simulink model "Copy_of_smlnk"  (R2024b)
settings: Solver=ode4  StartTime=0.0  StopTime=100  FixedStep=0.0001  RelTol=1e-3
model workspace (MAT data in the model file):
  Sample_Time = 0.0001
  Sig = Simulink.Signal
  Sig.Dimensions = -1
  Sig.DimensionsMode = 'auto'
  Sig.Complexity = 'auto'
  Sig.SampleTime = -1
  Sig.SamplingMode = 'auto'
  Sig.DataType = 'auto'
  Sig1 = Simulink.Signal
  Sig1.Dimensions = -1
  Sig1.DimensionsMode = 'auto'
  Sig1.Complexity = 'auto'
  Sig1.SampleTime = -1
  Sig1.SamplingMode = 'auto'
  Sig1.DataType = 'auto'
settings Model: Creator=loren  LastModifiedBy=loren
settings RTWCC: GPUComputeCapability=3.5
settings GRTTargetCC: RTWCAPISignals=on  RTWCAPIParams=on

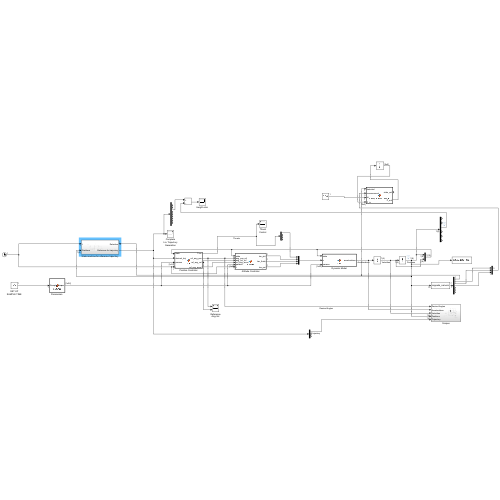
[thumbnail: Simulink's stored preview of the top-level diagram]
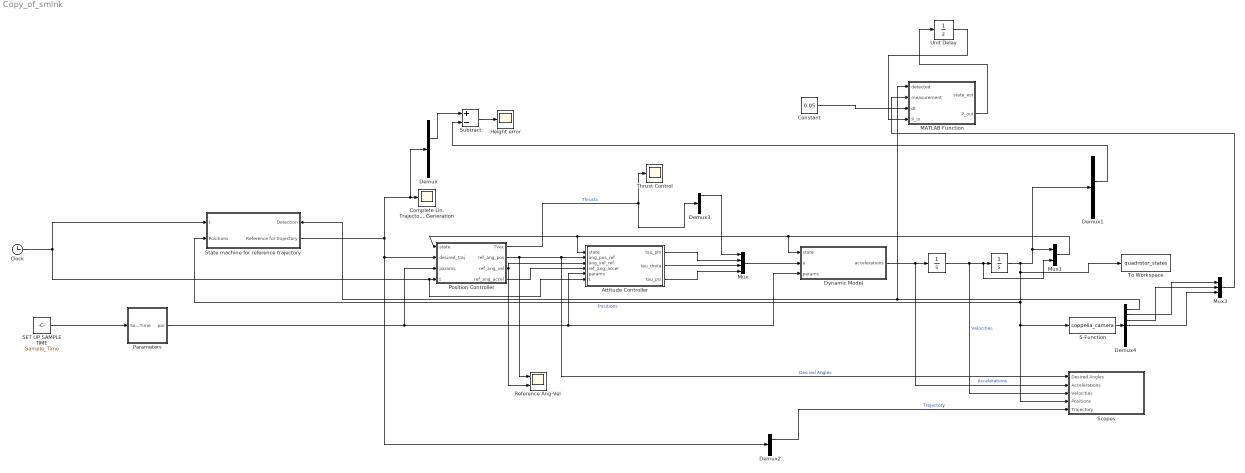
== system Copy_of_smlnk ==
  " " : Integrator  InitialCondition=[0 0 0 0 0 0]
  "  " : Integrator  InitialCondition=[0 0 0 0 0 0]
  Attitude Controller : MATLAB Function  TreatAsAtomicUnit=on  SystemSampleTime=Sample_Time
  Clock : Clock
  Complete Lin. Trajectory Generation : Scope
  Constant : Constant  Value=0.05
  Demux : Demux  Outputs=9
  Demux1 : Demux  Outputs=6
  Demux2 : Demux  Outputs=3
  Demux3 : Demux
  Demux4 : Demux  Outputs=7
  Dynamic Model : MATLAB Function  TreatAsAtomicUnit=on
  Height error : Scope
  MATLAB Function : MATLAB Function  TreatAsAtomicUnit=on
  Mux : Mux
  Mux1 : Mux  Inputs=2
  Mux3 : Mux  Inputs=3
  "Parameters " : MATLAB Function  TreatAsAtomicUnit=on  SystemSampleTime=Sample_Time
  Position Controller : MATLAB Function  TreatAsAtomicUnit=on  SystemSampleTime=Sample_Time
  Reference Ang-Vel : Scope  NumInputPorts=2
  S-Function : S-Function  FunctionName=coppelia_camera  Parameters=[Sample_Time, 1, 1]  SFunctionDeploymentMode=off  EnableBusSupport=off
  SET UP SAMPLE TIME : Constant  Value=Sample_Time
  Scopes : Subsystem
  State machine for reference trajectory : Subsystem
      settings: PortSchema="{\"entries\":[{\"content\":{\"sides\":[{\"content\":{\"connectorIds\":[\"In1\",\"In2\"]},\"type\":\"ConnectorPlacement.EquallySpacedRectSide\",\"uuid\":\"507c7cd5-8cc5-4e23-900b-3d7f1b18adf8\"},{\"content\":{\"connectorIds\":[\"In3\",\"Out1\"],\"side\":\"RIGHT\"},\"type\":\"ConnectorPlacement.EquallySpacedRectSide\",\"uuid\":\"450f9651-8ffa-4a7c-835b-1cc66628d75d\"},{\"content\":{\"side\":\"TOP\"},\"type\":\"ConnectorPlacement.EquallySpacedRectSide\",\"uuid\":\"2e914235-4cad-40eb-804a-8ecad3aa82e7\"}]},\"type\":\"ConnectorPlacement.EquallySpacedConnector\",\"uuid\":\"783284ba-16e5-4ade-a3ef-caf26ef0d258\"}],\"packageUris\":[\"http://schema.mathworks.com/mf0/Connector/R2020b\"],\"version\":\"1.0\"}"
  Subtract : Sum  Inputs=+-
  Thrust Control : Scope
  To Workspace : ToWorkspace  VariableName=quadrotor_states  SaveFormat=Structure With Time  SampleTime=-1
  Unit Delay : UnitDelay  InitialCondition=eye(5)  SampleTime=0.05  HasFrameUpgradeWarning=on
  wires:
  "Parameters "/1(par) -> Dynamic Model/3(params), Attitude Controller/5(params), Position Controller/3(params)
  Position Controller/2(ref_ang_pos) -> Reference Ang-Vel/1, Scopes/1(Desired Angles), Attitude Controller/2(ang_pos_ref)  "Desired Angles"
  Position Controller/3(ref_ang_vel) -> Reference Ang-Vel/2, Attitude Controller/3(ang_vel_ref)
  Attitude Controller/1(tau_phi) -> Mux/2
  Attitude Controller/2(tau_theta) -> Mux/3
  Attitude Controller/3(tau_psi) -> Mux/4
  Mux/1 -> Dynamic Model/2(u)
  Dynamic Model/1(accelerations) -> Scopes/2(Accelerations), " "/1  "Accelerations"
  " "/1 -> Scopes/3(Velocities), "  "/1, Mux1/2  "Velocities"
  Mux1/1 -> Dynamic Model/1(state), Position Controller/1(state), Attitude Controller/1(state)
  Demux/3 -> Subtract/1
  Demux1/3 -> Subtract/2
  Subtract/1 -> Height error/1
  Clock/1 -> Attitude Controller/6(t), Position Controller/4(t), State machine for reference trajectory/1(t)
  "  "/1 -> S-Function/1, Scopes/4(Positions), State machine for reference trajectory/2(Positions), To Workspace/1, Demux1/1, Mux1/1  "Positions"
  SET UP SAMPLE TIME/1 -> "Parameters "/1(Sample_Time)
  Position Controller/1(Tvec) -> Thrust Control/1, Demux3/1  "Thrusts"
  Demux3/1 -> Mux/1
  Demux2/1 -> Scopes/5(Trajectory)  "Trajectory"
  State machine for reference trajectory/1(Reference for trajectory) -> Demux/1, Complete Lin. Trajectory Generation/1, Position Controller/2(desired_traj), Demux2/1
  Position Controller/4(ref_ang_accel) -> Attitude Controller/4(ref_ang_accel)
  S-Function/1 -> Demux4/1
  Demux4/1 -> MATLAB Function/1(detected), State machine for reference trajectory/3(Detection)
  Demux4/2 -> Mux3/1
  Demux4/3 -> Mux3/2
  Demux4/4 -> Mux3/3
  Mux3/1 -> MATLAB Function/2(measurement)
  Constant/1 -> MATLAB Function/3(dt)
  MATLAB Function/2(P_out) -> Unit Delay/1
  Unit Delay/1 -> MATLAB Function/4(P_in)

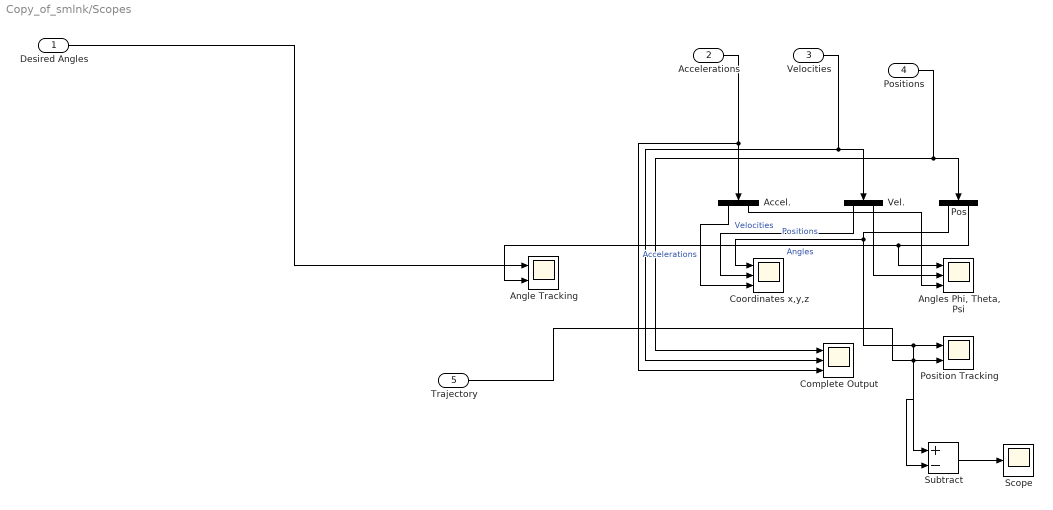
== system Copy_of_smlnk/Scopes ==
  Desired Angles : Inport
  Accelerations : Inport  Port=2
  Velocities : Inport  Port=3
  Positions : Inport  Port=4
  Trajectory : Inport  Port=5
  Accel. : Demux  Tag=Accelerations  Outputs=2
  Angle Tracking : Scope  NumInputPorts=2
  "Angles Phi, Theta, Psi" : Scope  NumInputPorts=3
  Complete Output : Scope  NumInputPorts=3
  Coordinates x,y,z : Scope  NumInputPorts=3
  Pos : Demux  Outputs=2
  Position Tracking : Scope  NumInputPorts=2
  Scope : Scope
  Subtract : Sum  Inputs=+-
  Vel. : Demux  Outputs=2
  wires:
  Accel./1 -> Coordinates x,y,z/3  "Accelerations"
  Pos/2 -> "Angles Phi, Theta, Psi"/1, Angle Tracking/2  "Angles"
  Accelerations/1 -> Accel./1, Complete Output/3
  Accel./2 -> "Angles Phi, Theta, Psi"/3
  Vel./2 -> "Angles Phi, Theta, Psi"/2
  Velocities/1 -> Vel./1, Complete Output/2
  Positions/1 -> Pos/1, Complete Output/1
  Pos/1 -> Subtract/1, Position Tracking/1, Coordinates x,y,z/1  "Positions"
  Vel./1 -> Coordinates x,y,z/2  "Velocities"
  Desired Angles/1 -> Angle Tracking/1
  Trajectory/1 -> Subtract/2, Position Tracking/2
  Subtract/1 -> Scope/1

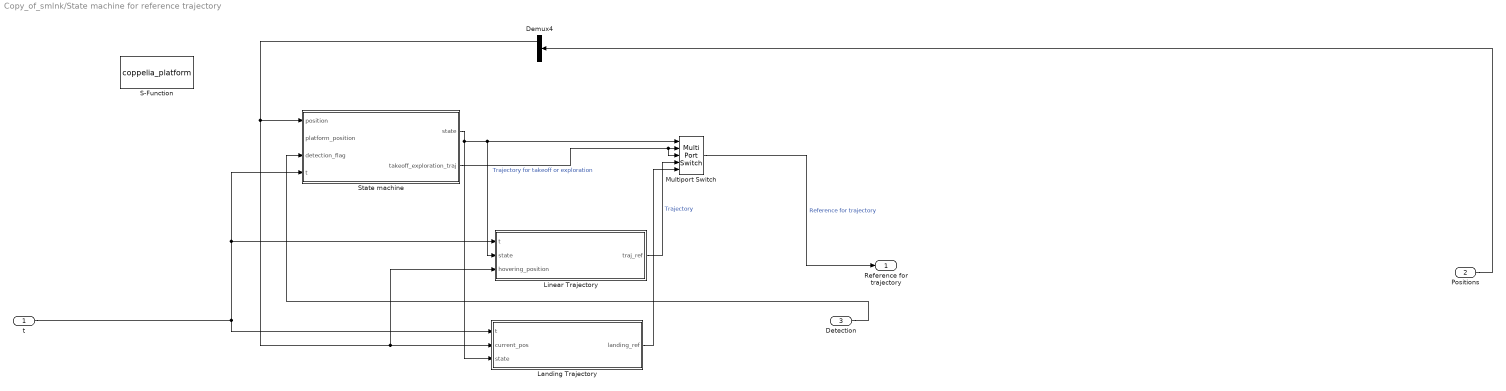
== system Copy_of_smlnk/State machine for reference trajectory ==
  t : Inport
  Positions : Inport  Port=2
  Detection : Inport  Port=3
  Demux4 : Demux  Outputs=2
  Landing Trajectory : MATLAB Function  TreatAsAtomicUnit=on  SystemSampleTime=Sample_Time
  Linear Trajectory : MATLAB Function  TreatAsAtomicUnit=on  SystemSampleTime=Sample_Time
  Multiport Switch : MultiPortSwitch  Inputs=4  SaturateOnIntegerOverflow=off  InputSameDT=off
  S-Function : S-Function  FunctionName=coppelia_platform  SFunctionDeploymentMode=off  EnableBusSupport=off
  State machine : MATLAB Function  TreatAsAtomicUnit=on  SystemSampleTime=Sample_Time
  Reference for trajectory : Outport
  wires:
  State machine/1(state) -> Landing Trajectory/3(state), Linear Trajectory/2(state), Multiport Switch/1
  t/1 -> Landing Trajectory/1(t), State machine/4(t), Linear Trajectory/1(t)
  Linear Trajectory/1(traj_ref) -> Multiport Switch/4  "Trajectory"
  Demux4/1 -> Linear Trajectory/3(hovering_position), Landing Trajectory/2(current_pos), State machine/1(position)
  Multiport Switch/1 -> Reference for trajectory/1  "Reference for trajectory"
  Positions/1 -> Demux4/1
  Landing Trajectory/1(landing_ref) -> Multiport Switch/5
  State machine/2(takeoff_exploration_traj) -> Multiport Switch/3, Multiport Switch/2  "Trajectory for takeoff or exploration"
  Detection/1 -> State machine/3(detection_flag)

== matlab function Copy_of_smlnk/State machine for reference trajectory/Linear Trajectory ==
  data: traj_ref output size=[1 9]; t input; state input; hovering_position input
function traj_ref = linear_trajectory(t,state,hovering_position)

% Chiama la funzione per generare la traiettoria
[pos, vel, acc] = only_linear_trajectory(t,hovering_position,state);
traj_ref = [pos, vel, acc];

== matlab function Copy_of_smlnk/Position Controller ==
  data: Tvec output; state input; desired_traj input; ref_ang_pos output; ref_ang_vel output; params input; t input; ref_ang_accel output
function [Tvec,ref_ang_pos,ref_ang_vel, ref_ang_accel] = pos(state,desired_traj,params,t)

[Tvec,ref_ang_pos,ref_ang_vel, ref_ang_accel] = position_control(desired_traj,state,params);

== matlab function Copy_of_smlnk/Parameters  ==
  data: par output; Sample_Time input
function par = params(Sample_Time)

[m,g,Ix,Iy,Iz,Kp_pos,Kd_pos,Ki_pos,Kp_ang,Kd_ang,Ki_ang,dt] = model_n_control_param();
%overwrites the Sample Time with the Environment sample time
dt=Sample_Time;
par = [m,g,Ix,Iy,Iz,Kp_pos,Kd_pos,Ki_pos,Kp_ang,Kd_ang,Ki_ang,dt];

== matlab function Copy_of_smlnk/Attitude Controller ==
  data: state input; ang_pos_ref input; tau_phi output size=1; ang_vel_ref input; ref_ang_accel input; params input; tau_theta output size=1; tau_psi output size=1; t input
function [tau_phi,tau_theta,tau_psi] = attitude(state,ang_pos_ref,ang_vel_ref,ref_ang_accel,params,t)

[tau_phi,tau_theta,tau_psi] = attitude_control(ang_pos_ref,ang_vel_ref,ref_ang_accel,state,params);

== matlab function Copy_of_smlnk/Dynamic Model ==
  data: state input; u input; accelerations output; params input
function accelerations = dyn(state,u,params)

accelerations = dynamic_model(state, u, params);

== matlab function Copy_of_smlnk/State machine for reference trajectory/State machine ==
  data: position input; state output; platform_position input; detection_flag input; t input; takeoff_exploration_traj output size=[1 9]
function [state, takeoff_exploration_traj]  = state_manager(position,platform_position,detection_flag,t)

[state, takeoff_exploration_traj] = stateManager(position,platform_position, detection_flag,t);

== matlab function Copy_of_smlnk/MATLAB Function ==
  data: detected input; state_est output; measurement input; dt input; P_in input; P_out output
function [state_est, P_out] = kalman_filter_block(detected, measurement, dt, P_in)
    [state_est, P_out] = kalman_filter_platform(detected, measurement, dt, P_in);
end

== matlab function Copy_of_smlnk/State machine for reference trajectory/Landing Trajectory ==
  data: t input; landing_ref output size=[1 9]; current_pos input size=[1 3]; state input
function landing_ref = landing_trajectory(t, current_pos, state)

[pos, vel, acc] = landing_trajectory(t, current_pos, state);
landing_ref = [pos, vel, acc];
